simulink model "Simple_Buck_BLDC_4_FaultModel"  (R2024a)
settings: Solver=VariableStepAuto  StartTime=0.0  StopTime=10.0  RelTol=1e-3  EnableMultiTasking=on
settings Model: Creator=feder  LastModifiedBy=feder
settings DebuggingCC: InheritedTsInSrcMsg=none

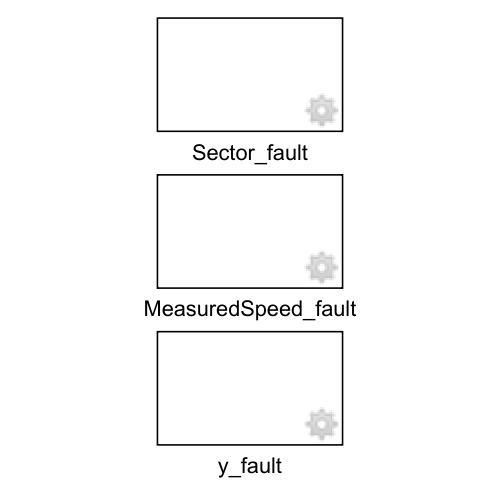
[thumbnail: Simulink's stored preview of the top-level diagram]
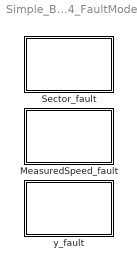
== system Simple_Buck_BLDC_4_FaultModel ==
  MeasuredSpeed_fault : Subsystem  TreatAsAtomicUnit=on  IsInjectorSS=on
      settings: LibrarySourceBlock=mwfaultlib/Stuck-at-Ground
  Sector_fault : Subsystem  TreatAsAtomicUnit=on  IsInjectorSS=on
      settings: LibrarySourceBlock=mwfaultlib/Stuck-at-Ground
  y_fault : Subsystem  TreatAsAtomicUnit=on  IsInjectorSS=on
      settings: LibrarySourceBlock=mwfaultlib/Stuck-at-Ground

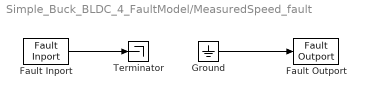
== system Simple_Buck_BLDC_4_FaultModel/MeasuredSpeed_fault ==
  Fault Inport : FaultInport
  Fault Outport : FaultOutport
  Ground : Ground
  Terminator : Terminator
  wires:
  Ground/1 -> Fault Outport/1
  Fault Inport/1 -> Terminator/1

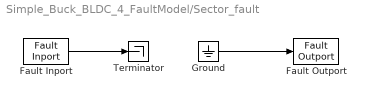
== system Simple_Buck_BLDC_4_FaultModel/Sector_fault ==
  Fault Inport : FaultInport
  Fault Outport : FaultOutport
  Ground : Ground
  Terminator : Terminator
  wires:
  Ground/1 -> Fault Outport/1
  Fault Inport/1 -> Terminator/1

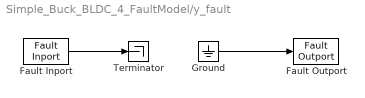
== system Simple_Buck_BLDC_4_FaultModel/y_fault ==
  Fault Inport : FaultInport
  Fault Outport : FaultOutport
  Ground : Ground
  Terminator : Terminator
  wires:
  Ground/1 -> Fault Outport/1
  Fault Inport/1 -> Terminator/1
